simulink model "TST_CoETS_StTrqLimCalc"  (R2016b)
settings: Solver=FixedStepDiscrete  StartTime=0.0  StopTime=simTime  FixedStep=sampleTime  RelTol=1e-3
values from neighbouring files (symbols this model uses):
  testCase = 1    [initTST_CoETS_StTrqLimCalc_001.m]    (also in initTST_CoETS_StTrqLimCalc_002.m = 2)
libraries: simulink x19, UnitTest_Lib x16
settings Model: Creator=zhengjinyan  LastModifiedBy=zhengjinyan
settings DebuggingCC: SignalRangeChecking=error

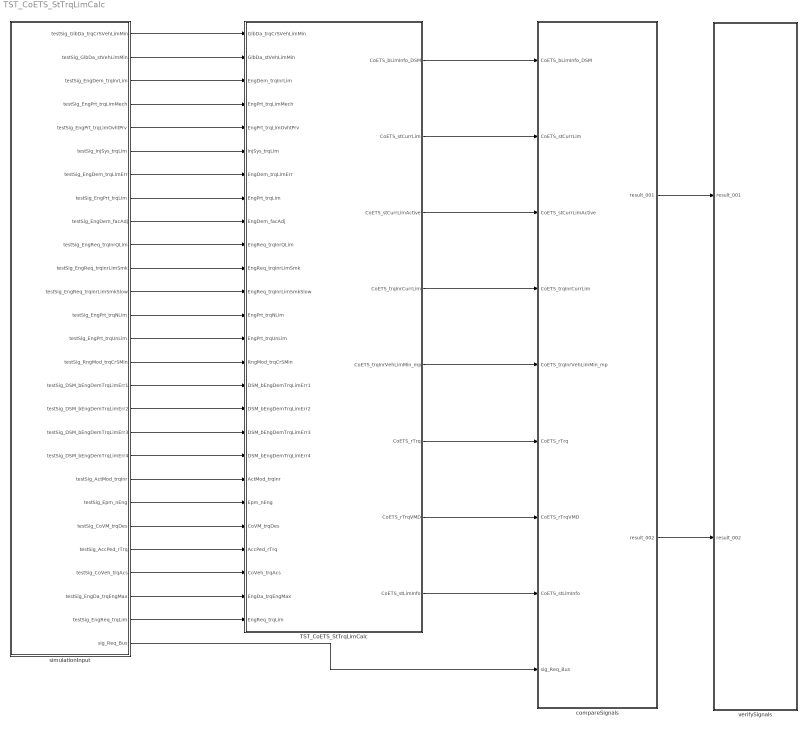
== system TST_CoETS_StTrqLimCalc ==
  TST_CoETS_StTrqLimCalc : Subsystem
  compareSignals : Subsystem
  simulationInput : Subsystem
  verifySignals : Subsystem
  wires:
  simulationInput/1(testSig_GlbDa_trqCrSVehLimMin) -> TST_CoETS_StTrqLimCalc/1(GlbDa_trqCrSVehLimMin)
  simulationInput/2(testSig_GlbDa_stVehLimMin) -> TST_CoETS_StTrqLimCalc/2(GlbDa_stVehLimMin)
  simulationInput/3(testSig_EngDem_trqInrLim) -> TST_CoETS_StTrqLimCalc/3(EngDem_trqInrLim)
  simulationInput/4(testSig_EngPrt_trqLimMech) -> TST_CoETS_StTrqLimCalc/4(EngPrt_trqLimMech)
  simulationInput/5(testSig_EngPrt_trqLimOvhtPrv) -> TST_CoETS_StTrqLimCalc/5(EngPrt_trqLimOvhtPrv)
  simulationInput/6(testSig_InjSys_trqLim) -> TST_CoETS_StTrqLimCalc/6(InjSys_trqLim)
  simulationInput/7(testSig_EngDem_trqLimErr) -> TST_CoETS_StTrqLimCalc/7(EngDem_trqLimErr)
  simulationInput/8(testSig_EngPrt_trqLim) -> TST_CoETS_StTrqLimCalc/8(EngPrt_trqLim)
  simulationInput/9(testSig_EngDem_facAdj) -> TST_CoETS_StTrqLimCalc/9(EngDem_facAdj)
  simulationInput/10(testSig_EngReq_trqInrQLim) -> TST_CoETS_StTrqLimCalc/10(EngReq_trqInrQLim)
  simulationInput/11(testSig_EngReq_trqInrLimSmk) -> TST_CoETS_StTrqLimCalc/11(EngReq_trqInrLimSmk)
  simulationInput/12(testSig_EngReq_trqInrLimSmkSlow) -> TST_CoETS_StTrqLimCalc/12(EngReq_trqInrLimSmkSlow)
  simulationInput/13(testSig_EngPrt_trqNLim) -> TST_CoETS_StTrqLimCalc/13(EngPrt_trqNLim)
  simulationInput/14(testSig_EngPrt_trqUnLim) -> TST_CoETS_StTrqLimCalc/14(EngPrt_trqUnLim)
  simulationInput/15(testSig_RngMod_trqCrSMin) -> TST_CoETS_StTrqLimCalc/15(RngMod_trqCrSMin)
  simulationInput/16(testSig_DSM_bEngDemTrqLimErr1) -> TST_CoETS_StTrqLimCalc/16(DSM_bEngDemTrqLimErr1)
  simulationInput/17(testSig_DSM_bEngDemTrqLimErr2) -> TST_CoETS_StTrqLimCalc/17(DSM_bEngDemTrqLimErr2)
  simulationInput/18(testSig_DSM_bEngDemTrqLimErr3) -> TST_CoETS_StTrqLimCalc/18(DSM_bEngDemTrqLimErr3)
  simulationInput/19(testSig_DSM_bEngDemTrqLimErr4) -> TST_CoETS_StTrqLimCalc/19(DSM_bEngDemTrqLimErr4)
  simulationInput/20(testSig_ActMod_trqInr) -> TST_CoETS_StTrqLimCalc/20(ActMod_trqInr)
  simulationInput/21(testSig_Epm_nEng) -> TST_CoETS_StTrqLimCalc/21(Epm_nEng)
  simulationInput/22(testSig_CoVM_trqDes) -> TST_CoETS_StTrqLimCalc/22(CoVM_trqDes)
  simulationInput/23(testSig_AccPed_rTrq) -> TST_CoETS_StTrqLimCalc/23(AccPed_rTrq)
  simulationInput/24(testSig_CoVeh_trqAcs) -> TST_CoETS_StTrqLimCalc/24(CoVeh_trqAcs)
  simulationInput/25(testSig_EngDa_trqEngMax) -> TST_CoETS_StTrqLimCalc/25(EngDa_trqEngMax)
  simulationInput/26(testSig_EngReq_trqLim) -> TST_CoETS_StTrqLimCalc/26(EngReq_trqLim)
  TST_CoETS_StTrqLimCalc/1(CoETS_bLimInfo_DSM) -> compareSignals/1(CoETS_bLimInfo_DSM)
  TST_CoETS_StTrqLimCalc/2(CoETS_stCurrLim) -> compareSignals/2(CoETS_stCurrLim)
  TST_CoETS_StTrqLimCalc/3(CoETS_stCurrLimActive) -> compareSignals/3(CoETS_stCurrLimActive)
  TST_CoETS_StTrqLimCalc/4(CoETS_trqInrCurrLim) -> compareSignals/4(CoETS_trqInrCurrLim)
  TST_CoETS_StTrqLimCalc/5(CoETS_trqInrVehLimMin_mp) -> compareSignals/5(CoETS_trqInrVehLimMin_mp)
  TST_CoETS_StTrqLimCalc/6(CoETS_rTrq) -> compareSignals/6(CoETS_rTrq)
  TST_CoETS_StTrqLimCalc/7(CoETS_rTrqVMD) -> compareSignals/7(CoETS_rTrqVMD)
  TST_CoETS_StTrqLimCalc/8(CoETS_stLimInfo) -> compareSignals/8(CoETS_stLimInfo)
  simulationInput/27(sig_Req_Bus) -> compareSignals/9(sig_Req_Bus)
  compareSignals/1(result_001) -> verifySignals/1(result_001)
  compareSignals/2(result_002) -> verifySignals/2(result_002)

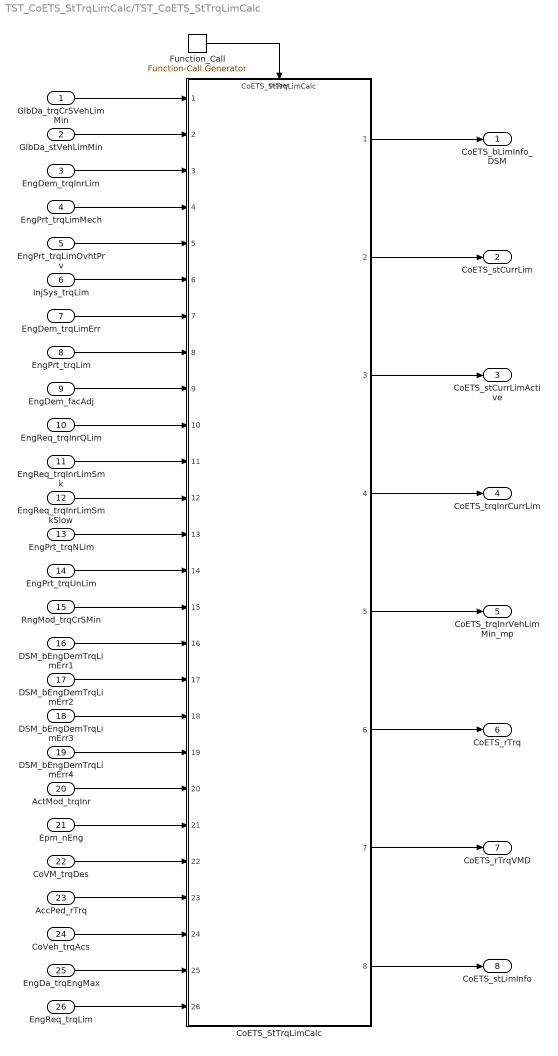
== system TST_CoETS_StTrqLimCalc/TST_CoETS_StTrqLimCalc ==
  GlbDa_trqCrSVehLimMin : Inport
  GlbDa_stVehLimMin : Inport  Port=2
  EngDem_trqInrLim : Inport  Port=3
  EngPrt_trqLimMech : Inport  Port=4
  EngPrt_trqLimOvhtPrv : Inport  Port=5
  InjSys_trqLim : Inport  Port=6
  EngDem_trqLimErr : Inport  Port=7
  EngPrt_trqLim : Inport  Port=8
  EngDem_facAdj : Inport  Port=9
  EngReq_trqInrQLim : Inport  Port=10
  EngReq_trqInrLimSmk : Inport  Port=11
  EngReq_trqInrLimSmkSlow : Inport  Port=12
  EngPrt_trqNLim : Inport  Port=13
  EngPrt_trqUnLim : Inport  Port=14
  RngMod_trqCrSMin : Inport  Port=15
  DSM_bEngDemTrqLimErr1 : Inport  Port=16
  DSM_bEngDemTrqLimErr2 : Inport  Port=17
  DSM_bEngDemTrqLimErr3 : Inport  Port=18
  DSM_bEngDemTrqLimErr4 : Inport  Port=19
  ActMod_trqInr : Inport  Port=20
  Epm_nEng : Inport  Port=21
  CoVM_trqDes : Inport  Port=22
  AccPed_rTrq : Inport  Port=23
  CoVeh_trqAcs : Inport  Port=24
  EngDa_trqEngMax : Inport  Port=25
  EngReq_trqLim : Inport  Port=26
  CoETS_StTrqLimCalc : ModelReference  ModelNameDialog=CoETS_StTrqLimCalc  SimulationMode=Normal  ModelReferenceVersion=1.4  TriggerPortName=function  TriggerPortTriggerType=function-call  TriggerPortStatesWhenEnabling=held
  Function_Call : simulink/Ports & Subsystems/Function-Call Generator  sample_time=sampleTime  numberOfIterations=1
  CoETS_bLimInfo_DSM : Outport
  CoETS_stCurrLim : Outport  Port=2
  CoETS_stCurrLimActive : Outport  Port=3
  CoETS_trqInrCurrLim : Outport  Port=4
  CoETS_trqInrVehLimMin_mp : Outport  Port=5
  CoETS_rTrq : Outport  Port=6
  CoETS_rTrqVMD : Outport  Port=7
  CoETS_stLimInfo : Outport  Port=8
  wires:
  Function_Call/1 -> CoETS_StTrqLimCalc/Trigger
  GlbDa_trqCrSVehLimMin/1 -> CoETS_StTrqLimCalc/1
  GlbDa_stVehLimMin/1 -> CoETS_StTrqLimCalc/2
  EngDem_trqInrLim/1 -> CoETS_StTrqLimCalc/3
  EngPrt_trqLimMech/1 -> CoETS_StTrqLimCalc/4
  EngPrt_trqLimOvhtPrv/1 -> CoETS_StTrqLimCalc/5
  InjSys_trqLim/1 -> CoETS_StTrqLimCalc/6
  EngDem_trqLimErr/1 -> CoETS_StTrqLimCalc/7
  EngPrt_trqLim/1 -> CoETS_StTrqLimCalc/8
  EngDem_facAdj/1 -> CoETS_StTrqLimCalc/9
  EngReq_trqInrQLim/1 -> CoETS_StTrqLimCalc/10
  EngReq_trqInrLimSmk/1 -> CoETS_StTrqLimCalc/11
  EngReq_trqInrLimSmkSlow/1 -> CoETS_StTrqLimCalc/12
  EngPrt_trqNLim/1 -> CoETS_StTrqLimCalc/13
  EngPrt_trqUnLim/1 -> CoETS_StTrqLimCalc/14
  RngMod_trqCrSMin/1 -> CoETS_StTrqLimCalc/15
  DSM_bEngDemTrqLimErr1/1 -> CoETS_StTrqLimCalc/16
  DSM_bEngDemTrqLimErr2/1 -> CoETS_StTrqLimCalc/17
  DSM_bEngDemTrqLimErr3/1 -> CoETS_StTrqLimCalc/18
  DSM_bEngDemTrqLimErr4/1 -> CoETS_StTrqLimCalc/19
  ActMod_trqInr/1 -> CoETS_StTrqLimCalc/20
  Epm_nEng/1 -> CoETS_StTrqLimCalc/21
  CoVM_trqDes/1 -> CoETS_StTrqLimCalc/22
  AccPed_rTrq/1 -> CoETS_StTrqLimCalc/23
  CoVeh_trqAcs/1 -> CoETS_StTrqLimCalc/24
  EngDa_trqEngMax/1 -> CoETS_StTrqLimCalc/25
  EngReq_trqLim/1 -> CoETS_StTrqLimCalc/26
  CoETS_StTrqLimCalc/1 -> CoETS_bLimInfo_DSM/1
  CoETS_StTrqLimCalc/2 -> CoETS_stCurrLim/1
  CoETS_StTrqLimCalc/3 -> CoETS_stCurrLimActive/1
  CoETS_StTrqLimCalc/4 -> CoETS_trqInrCurrLim/1
  CoETS_StTrqLimCalc/5 -> CoETS_trqInrVehLimMin_mp/1
  CoETS_StTrqLimCalc/6 -> CoETS_rTrq/1
  CoETS_StTrqLimCalc/7 -> CoETS_rTrqVMD/1
  CoETS_StTrqLimCalc/8 -> CoETS_stLimInfo/1

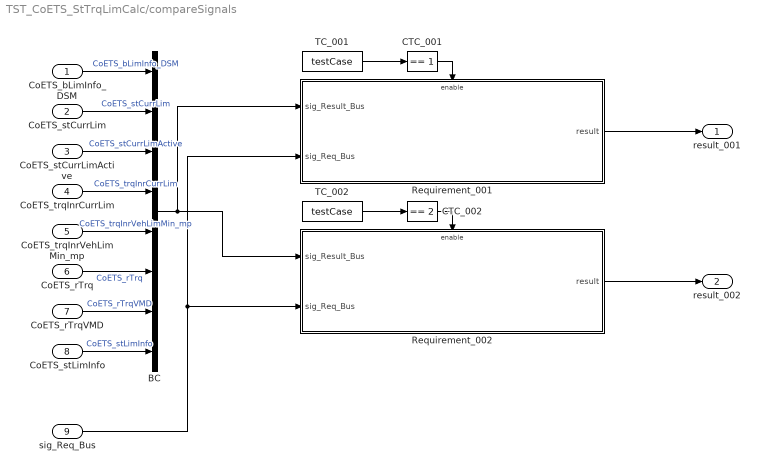
== system TST_CoETS_StTrqLimCalc/compareSignals ==
  CoETS_bLimInfo_DSM : Inport
  CoETS_stCurrLim : Inport  Port=2
  CoETS_stCurrLimActive : Inport  Port=3
  CoETS_trqInrCurrLim : Inport  Port=4
  CoETS_trqInrVehLimMin_mp : Inport  Port=5
  CoETS_rTrq : Inport  Port=6
  CoETS_rTrqVMD : Inport  Port=7
  CoETS_stLimInfo : Inport  Port=8
  sig_Req_Bus : Inport  Port=9
  BC : BusCreator  Inputs=8
  CTC_001 : simulink/Logic and Bit Operations/Compare To Constant  relop===  const=1  OutDataTypeStr=boolean
  CTC_002 : simulink/Logic and Bit Operations/Compare To Constant  relop===  const=2  OutDataTypeStr=boolean
  Requirement_001 : Subsystem
  Requirement_002 : Subsystem
  TC_001 : Constant  Value=testCase
  TC_002 : Constant  Value=testCase
  result_001 : Outport
  result_002 : Outport  Port=2
  wires:
  CoETS_bLimInfo_DSM/1 -> BC/1  "CoETS_bLimInfo_DSM"
  CoETS_stCurrLim/1 -> BC/2  "CoETS_stCurrLim"
  CoETS_stCurrLimActive/1 -> BC/3  "CoETS_stCurrLimActive"
  CoETS_trqInrCurrLim/1 -> BC/4  "CoETS_trqInrCurrLim"
  CoETS_trqInrVehLimMin_mp/1 -> BC/5  "CoETS_trqInrVehLimMin_mp"
  CoETS_rTrq/1 -> BC/6  "CoETS_rTrq"
  CoETS_rTrqVMD/1 -> BC/7  "CoETS_rTrqVMD"
  CoETS_stLimInfo/1 -> BC/8  "CoETS_stLimInfo"
  TC_001/1 -> CTC_001/1
  CTC_001/1 -> Requirement_001/Enable
  sig_Req_Bus/1 -> Requirement_001/2(sig_Req_Bus), Requirement_002/2(sig_Req_Bus)
  BC/1 -> Requirement_001/1(sig_Result_Bus), Requirement_002/1(sig_Result_Bus)
  Requirement_001/1(result) -> result_001/1
  TC_002/1 -> CTC_002/1
  CTC_002/1 -> Requirement_002/Enable
  Requirement_002/1(result) -> result_002/1

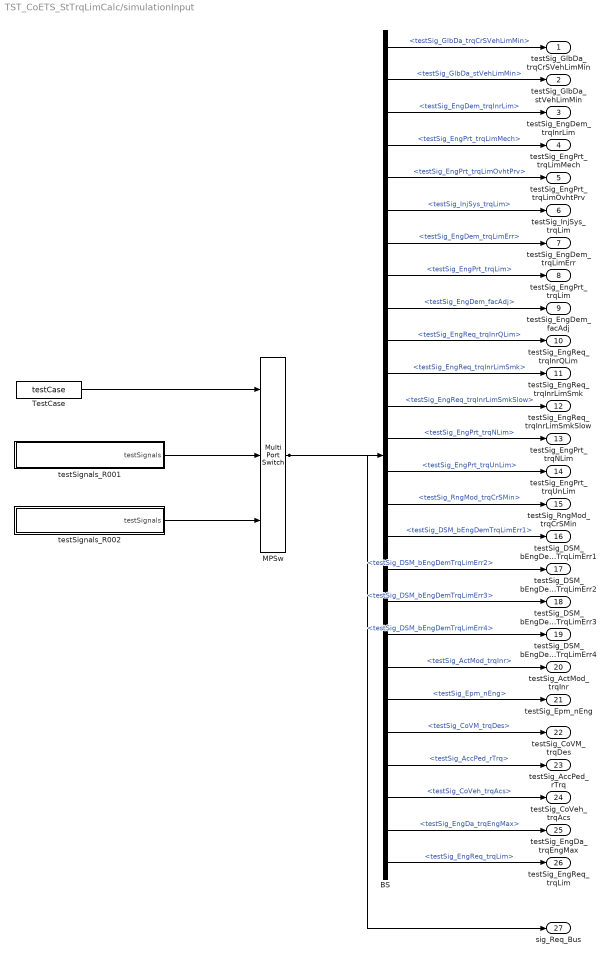
== system TST_CoETS_StTrqLimCalc/simulationInput ==
  BS : BusSelector  OutputSignals=testSig_GlbDa_trqCrSVehLimMin,testSig_GlbDa_stVehLimMin,testSig_EngDem_trqInrLim,testSig_EngPrt_trqLimMech,testSig_EngPrt_trqLimOvhtPrv,testSig_InjSys_trqLim,testSig_EngDem_trqLimErr,testSig_EngPrt_trqLim,testSig_EngDem_facAdj,testSig_EngReq_trqInrQLim,testSig_EngReq_trqInrLimSmk,testSig_EngReq_trqInrLimSmkSlow,testSig_EngPrt_trqNLim,testSig_EngPrt_trqUnLim,testSig_RngMod_trqCrSMin,testSig_DSM_bEngDemTrqLimErr1,testSig_DSM_bEngDemTrqLimErr2,testSig_DSM_bEngDemTrqLimErr3,testSig_DSM_bEngDemTrqLimErr4,testSig_ActMod_trqInr,testSig_Epm_nEng,testSig_CoVM_trqDes,testSig_AccPed_rTrq,testSig_CoVeh_trqAcs,testSig_EngDa_trqEngMax,testSig_EngReq_trqLim
  MPSw : MultiPortSwitch  Inputs=2  SaturateOnIntegerOverflow=on  InputSameDT=on
  TestCase : Constant  Value=testCase
  testSignals_R001 : Subsystem
  testSignals_R002 : Subsystem
  testSig_GlbDa_trqCrSVehLimMin : Outport
  testSig_GlbDa_stVehLimMin : Outport  Port=2
  testSig_EngDem_trqInrLim : Outport  Port=3
  testSig_EngPrt_trqLimMech : Outport  Port=4
  testSig_EngPrt_trqLimOvhtPrv : Outport  Port=5
  testSig_InjSys_trqLim : Outport  Port=6
  testSig_EngDem_trqLimErr : Outport  Port=7
  testSig_EngPrt_trqLim : Outport  Port=8
  testSig_EngDem_facAdj : Outport  Port=9
  testSig_EngReq_trqInrQLim : Outport  Port=10
  testSig_EngReq_trqInrLimSmk : Outport  Port=11
  testSig_EngReq_trqInrLimSmkSlow : Outport  Port=12
  testSig_EngPrt_trqNLim : Outport  Port=13
  testSig_EngPrt_trqUnLim : Outport  Port=14
  testSig_RngMod_trqCrSMin : Outport  Port=15
  testSig_DSM_bEngDemTrqLimErr1 : Outport  Port=16
  testSig_DSM_bEngDemTrqLimErr2 : Outport  Port=17
  testSig_DSM_bEngDemTrqLimErr3 : Outport  Port=18
  testSig_DSM_bEngDemTrqLimErr4 : Outport  Port=19
  testSig_ActMod_trqInr : Outport  Port=20
  testSig_Epm_nEng : Outport  Port=21
  testSig_CoVM_trqDes : Outport  Port=22
  testSig_AccPed_rTrq : Outport  Port=23
  testSig_CoVeh_trqAcs : Outport  Port=24
  testSig_EngDa_trqEngMax : Outport  Port=25
  testSig_EngReq_trqLim : Outport  Port=26
  sig_Req_Bus : Outport  Port=27
  wires:
  BS/1 -> testSig_GlbDa_trqCrSVehLimMin/1  "<testSig_GlbDa_trqCrSVehLimMin>"
  BS/2 -> testSig_GlbDa_stVehLimMin/1  "<testSig_GlbDa_stVehLimMin>"
  BS/3 -> testSig_EngDem_trqInrLim/1  "<testSig_EngDem_trqInrLim>"
  BS/4 -> testSig_EngPrt_trqLimMech/1  "<testSig_EngPrt_trqLimMech>"
  BS/5 -> testSig_EngPrt_trqLimOvhtPrv/1  "<testSig_EngPrt_trqLimOvhtPrv>"
  BS/6 -> testSig_InjSys_trqLim/1  "<testSig_InjSys_trqLim>"
  BS/7 -> testSig_EngDem_trqLimErr/1  "<testSig_EngDem_trqLimErr>"
  BS/8 -> testSig_EngPrt_trqLim/1  "<testSig_EngPrt_trqLim>"
  BS/9 -> testSig_EngDem_facAdj/1  "<testSig_EngDem_facAdj>"
  BS/10 -> testSig_EngReq_trqInrQLim/1  "<testSig_EngReq_trqInrQLim>"
  BS/11 -> testSig_EngReq_trqInrLimSmk/1  "<testSig_EngReq_trqInrLimSmk>"
  BS/12 -> testSig_EngReq_trqInrLimSmkSlow/1  "<testSig_EngReq_trqInrLimSmkSlow>"
  BS/13 -> testSig_EngPrt_trqNLim/1  "<testSig_EngPrt_trqNLim>"
  BS/14 -> testSig_EngPrt_trqUnLim/1  "<testSig_EngPrt_trqUnLim>"
  BS/15 -> testSig_RngMod_trqCrSMin/1  "<testSig_RngMod_trqCrSMin>"
  BS/16 -> testSig_DSM_bEngDemTrqLimErr1/1  "<testSig_DSM_bEngDemTrqLimErr1>"
  BS/17 -> testSig_DSM_bEngDemTrqLimErr2/1  "<testSig_DSM_bEngDemTrqLimErr2>"
  BS/18 -> testSig_DSM_bEngDemTrqLimErr3/1  "<testSig_DSM_bEngDemTrqLimErr3>"
  BS/19 -> testSig_DSM_bEngDemTrqLimErr4/1  "<testSig_DSM_bEngDemTrqLimErr4>"
  BS/20 -> testSig_ActMod_trqInr/1  "<testSig_ActMod_trqInr>"
  BS/21 -> testSig_Epm_nEng/1  "<testSig_Epm_nEng>"
  BS/22 -> testSig_CoVM_trqDes/1  "<testSig_CoVM_trqDes>"
  BS/23 -> testSig_AccPed_rTrq/1  "<testSig_AccPed_rTrq>"
  BS/24 -> testSig_CoVeh_trqAcs/1  "<testSig_CoVeh_trqAcs>"
  BS/25 -> testSig_EngDa_trqEngMax/1  "<testSig_EngDa_trqEngMax>"
  BS/26 -> testSig_EngReq_trqLim/1  "<testSig_EngReq_trqLim>"
  MPSw/1 -> BS/1, sig_Req_Bus/1
  TestCase/1 -> MPSw/1
  testSignals_R001/1(testSignals) -> MPSw/2
  testSignals_R002/1(testSignals) -> MPSw/3

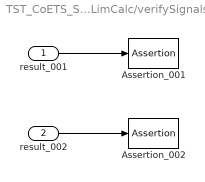
== system TST_CoETS_StTrqLimCalc/verifySignals ==
  result_001 : Inport
  result_002 : Inport  Port=2
  Assertion_001 : Assertion  Enabled=off
  Assertion_002 : Assertion  Enabled=off
  wires:
  result_001/1 -> Assertion_001/1
  result_002/1 -> Assertion_002/1

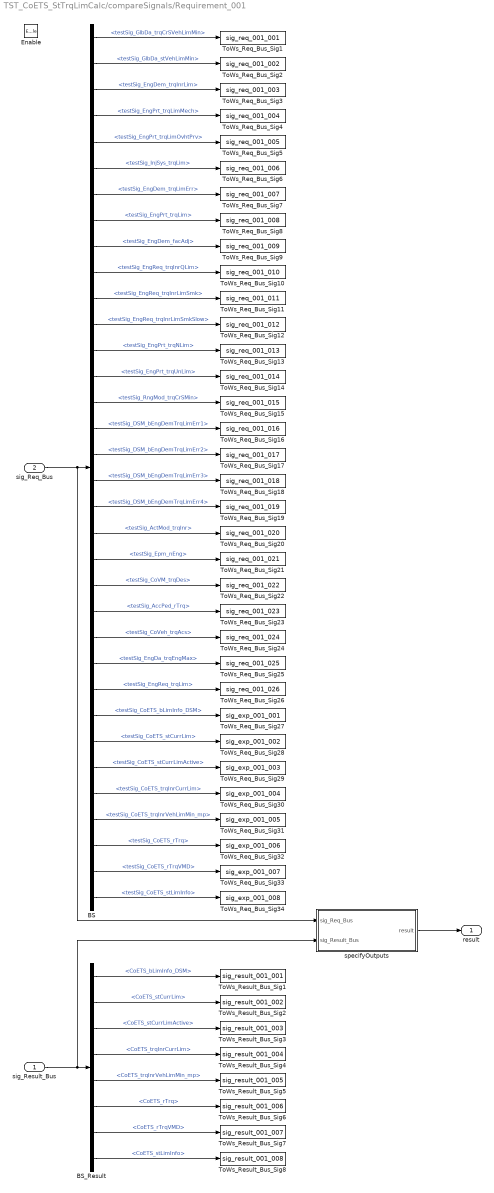
== system TST_CoETS_StTrqLimCalc/compareSignals/Requirement_001 ==
  sig_Result_Bus : Inport
  sig_Req_Bus : Inport  Port=2
  Enable : EnablePort
  BS : BusSelector  OutputSignals=testSig_GlbDa_trqCrSVehLimMin,testSig_GlbDa_stVehLimMin,testSig_EngDem_trqInrLim,testSig_EngPrt_trqLimMech,testSig_EngPrt_trqLimOvhtPrv,testSig_InjSys_trqLim,testSig_EngDem_trqLimErr,testSig_EngPrt_trqLim,testSig_EngDem_facAdj,testSig_EngReq_trqInrQLim,testSig_EngReq_trqInrLimSmk,testSig_EngReq_trqInrLimSmkSlow,testSig_EngPrt_trqNLim,testSig_EngPrt_trqUnLim,testSig_RngMod_trqCrSMin,testSig_DSM_bEngDemTrqLimErr1,testSig_DSM_bEngDemTrqLimErr2,testSig_DSM_bEngDemTrqLimErr3,testSig_DSM_bEngDemTrqLimErr4,testSig_ActMod_trqInr,testSig_Epm_nEng,testSig_CoVM_trqDes,testSig_AccPed_rTrq,testSig_CoVeh_trqAcs,testSig_EngDa_trqEngMax,testSig_EngReq_trqLim,testSig_CoETS_bLimInfo_DSM,testSig_CoETS_stCurrLim,testSig_CoETS_stCurrLimActive,testSig_CoETS_trqInrCurrLim,testSig_CoETS_trqInrVehLimMin_mp,testSig_CoETS_rTrq,testSig_CoETS_rTrqVMD,testSig_CoETS_stLimInfo
  BS_Result : BusSelector  OutputSignals=CoETS_bLimInfo_DSM,CoETS_stCurrLim,CoETS_stCurrLimActive,CoETS_trqInrCurrLim,CoETS_trqInrVehLimMin_mp,CoETS_rTrq,CoETS_rTrqVMD,CoETS_stLimInfo
  ToWs_Req_Bus_Sig1 : ToWorkspace  VariableName=sig_req_001_001  SaveFormat=Structure With Time
  ToWs_Req_Bus_Sig10 : ToWorkspace  VariableName=sig_req_001_010  SaveFormat=Structure With Time
  ToWs_Req_Bus_Sig11 : ToWorkspace  VariableName=sig_req_001_011  SaveFormat=Structure With Time
  ToWs_Req_Bus_Sig12 : ToWorkspace  VariableName=sig_req_001_012  SaveFormat=Structure With Time
  ToWs_Req_Bus_Sig13 : ToWorkspace  VariableName=sig_req_001_013  SaveFormat=Structure With Time
  ToWs_Req_Bus_Sig14 : ToWorkspace  VariableName=sig_req_001_014  SaveFormat=Structure With Time
  ToWs_Req_Bus_Sig15 : ToWorkspace  VariableName=sig_req_001_015  SaveFormat=Structure With Time
  ToWs_Req_Bus_Sig16 : ToWorkspace  VariableName=sig_req_001_016  SaveFormat=Structure With Time
  ToWs_Req_Bus_Sig17 : ToWorkspace  VariableName=sig_req_001_017  SaveFormat=Structure With Time
  ToWs_Req_Bus_Sig18 : ToWorkspace  VariableName=sig_req_001_018  SaveFormat=Structure With Time
  ToWs_Req_Bus_Sig19 : ToWorkspace  VariableName=sig_req_001_019  SaveFormat=Structure With Time
  ToWs_Req_Bus_Sig2 : ToWorkspace  VariableName=sig_req_001_002  SaveFormat=Structure With Time
  ToWs_Req_Bus_Sig20 : ToWorkspace  VariableName=sig_req_001_020  SaveFormat=Structure With Time
  ToWs_Req_Bus_Sig21 : ToWorkspace  VariableName=sig_req_001_021  SaveFormat=Structure With Time
  ToWs_Req_Bus_Sig22 : ToWorkspace  VariableName=sig_req_001_022  SaveFormat=Structure With Time
  ToWs_Req_Bus_Sig23 : ToWorkspace  VariableName=sig_req_001_023  SaveFormat=Structure With Time
  ToWs_Req_Bus_Sig24 : ToWorkspace  VariableName=sig_req_001_024  SaveFormat=Structure With Time
  ToWs_Req_Bus_Sig25 : ToWorkspace  VariableName=sig_req_001_025  SaveFormat=Structure With Time
  ToWs_Req_Bus_Sig26 : ToWorkspace  VariableName=sig_req_001_026  SaveFormat=Structure With Time
  ToWs_Req_Bus_Sig27 : ToWorkspace  VariableName=sig_exp_001_001  SaveFormat=Structure With Time
  ToWs_Req_Bus_Sig28 : ToWorkspace  VariableName=sig_exp_001_002  SaveFormat=Structure With Time
  ToWs_Req_Bus_Sig29 : ToWorkspace  VariableName=sig_exp_001_003  SaveFormat=Structure With Time
  ToWs_Req_Bus_Sig3 : ToWorkspace  VariableName=sig_req_001_003  SaveFormat=Structure With Time
  ToWs_Req_Bus_Sig30 : ToWorkspace  VariableName=sig_exp_001_004  SaveFormat=Structure With Time
  ToWs_Req_Bus_Sig31 : ToWorkspace  VariableName=sig_exp_001_005  SaveFormat=Structure With Time
  ToWs_Req_Bus_Sig32 : ToWorkspace  VariableName=sig_exp_001_006  SaveFormat=Structure With Time
  ToWs_Req_Bus_Sig33 : ToWorkspace  VariableName=sig_exp_001_007  SaveFormat=Structure With Time
  ToWs_Req_Bus_Sig34 : ToWorkspace  VariableName=sig_exp_001_008  SaveFormat=Structure With Time
  ToWs_Req_Bus_Sig4 : ToWorkspace  VariableName=sig_req_001_004  SaveFormat=Structure With Time
  ToWs_Req_Bus_Sig5 : ToWorkspace  VariableName=sig_req_001_005  SaveFormat=Structure With Time
  ToWs_Req_Bus_Sig6 : ToWorkspace  VariableName=sig_req_001_006  SaveFormat=Structure With Time
  ToWs_Req_Bus_Sig7 : ToWorkspace  VariableName=sig_req_001_007  SaveFormat=Structure With Time
  ToWs_Req_Bus_Sig8 : ToWorkspace  VariableName=sig_req_001_008  SaveFormat=Structure With Time
  ToWs_Req_Bus_Sig9 : ToWorkspace  VariableName=sig_req_001_009  SaveFormat=Structure With Time
  ToWs_Result_Bus_Sig1 : ToWorkspace  VariableName=sig_result_001_001  SaveFormat=Structure With Time
  ToWs_Result_Bus_Sig2 : ToWorkspace  VariableName=sig_result_001_002  SaveFormat=Structure With Time
  ToWs_Result_Bus_Sig3 : ToWorkspace  VariableName=sig_result_001_003  SaveFormat=Structure With Time
  ToWs_Result_Bus_Sig4 : ToWorkspace  VariableName=sig_result_001_004  SaveFormat=Structure With Time
  ToWs_Result_Bus_Sig5 : ToWorkspace  VariableName=sig_result_001_005  SaveFormat=Structure With Time
  ToWs_Result_Bus_Sig6 : ToWorkspace  VariableName=sig_result_001_006  SaveFormat=Structure With Time
  ToWs_Result_Bus_Sig7 : ToWorkspace  VariableName=sig_result_001_007  SaveFormat=Structure With Time
  ToWs_Result_Bus_Sig8 : ToWorkspace  VariableName=sig_result_001_008  SaveFormat=Structure With Time
  specifyOutputs : Subsystem
  result : Outport
  wires:
  sig_Req_Bus/1 -> BS/1, specifyOutputs/1(sig_Req_Bus)
  BS/1 -> ToWs_Req_Bus_Sig1/1  "<testSig_GlbDa_trqCrSVehLimMin>"
  BS/2 -> ToWs_Req_Bus_Sig2/1  "<testSig_GlbDa_stVehLimMin>"
  BS/3 -> ToWs_Req_Bus_Sig3/1  "<testSig_EngDem_trqInrLim>"
  BS/4 -> ToWs_Req_Bus_Sig4/1  "<testSig_EngPrt_trqLimMech>"
  BS/5 -> ToWs_Req_Bus_Sig5/1  "<testSig_EngPrt_trqLimOvhtPrv>"
  BS/6 -> ToWs_Req_Bus_Sig6/1  "<testSig_InjSys_trqLim>"
  BS/7 -> ToWs_Req_Bus_Sig7/1  "<testSig_EngDem_trqLimErr>"
  BS/8 -> ToWs_Req_Bus_Sig8/1  "<testSig_EngPrt_trqLim>"
  BS/9 -> ToWs_Req_Bus_Sig9/1  "<testSig_EngDem_facAdj>"
  BS/10 -> ToWs_Req_Bus_Sig10/1  "<testSig_EngReq_trqInrQLim>"
  BS/11 -> ToWs_Req_Bus_Sig11/1  "<testSig_EngReq_trqInrLimSmk>"
  BS/12 -> ToWs_Req_Bus_Sig12/1  "<testSig_EngReq_trqInrLimSmkSlow>"
  BS/13 -> ToWs_Req_Bus_Sig13/1  "<testSig_EngPrt_trqNLim>"
  BS/14 -> ToWs_Req_Bus_Sig14/1  "<testSig_EngPrt_trqUnLim>"
  BS/15 -> ToWs_Req_Bus_Sig15/1  "<testSig_RngMod_trqCrSMin>"
  BS/16 -> ToWs_Req_Bus_Sig16/1  "<testSig_DSM_bEngDemTrqLimErr1>"
  BS/17 -> ToWs_Req_Bus_Sig17/1  "<testSig_DSM_bEngDemTrqLimErr2>"
  BS/18 -> ToWs_Req_Bus_Sig18/1  "<testSig_DSM_bEngDemTrqLimErr3>"
  BS/19 -> ToWs_Req_Bus_Sig19/1  "<testSig_DSM_bEngDemTrqLimErr4>"
  BS/20 -> ToWs_Req_Bus_Sig20/1  "<testSig_ActMod_trqInr>"
  BS/21 -> ToWs_Req_Bus_Sig21/1  "<testSig_Epm_nEng>"
  BS/22 -> ToWs_Req_Bus_Sig22/1  "<testSig_CoVM_trqDes>"
  BS/23 -> ToWs_Req_Bus_Sig23/1  "<testSig_AccPed_rTrq>"
  BS/24 -> ToWs_Req_Bus_Sig24/1  "<testSig_CoVeh_trqAcs>"
  BS/25 -> ToWs_Req_Bus_Sig25/1  "<testSig_EngDa_trqEngMax>"
  BS/26 -> ToWs_Req_Bus_Sig26/1  "<testSig_EngReq_trqLim>"
  BS/27 -> ToWs_Req_Bus_Sig27/1  "<testSig_CoETS_bLimInfo_DSM>"
  BS/28 -> ToWs_Req_Bus_Sig28/1  "<testSig_CoETS_stCurrLim>"
  BS/29 -> ToWs_Req_Bus_Sig29/1  "<testSig_CoETS_stCurrLimActive>"
  BS/30 -> ToWs_Req_Bus_Sig30/1  "<testSig_CoETS_trqInrCurrLim>"
  BS/31 -> ToWs_Req_Bus_Sig31/1  "<testSig_CoETS_trqInrVehLimMin_mp>"
  BS/32 -> ToWs_Req_Bus_Sig32/1  "<testSig_CoETS_rTrq>"
  BS/33 -> ToWs_Req_Bus_Sig33/1  "<testSig_CoETS_rTrqVMD>"
  BS/34 -> ToWs_Req_Bus_Sig34/1  "<testSig_CoETS_stLimInfo>"
  sig_Result_Bus/1 -> BS_Result/1, specifyOutputs/2(sig_Result_Bus)
  BS_Result/1 -> ToWs_Result_Bus_Sig1/1  "<CoETS_bLimInfo_DSM>"
  BS_Result/2 -> ToWs_Result_Bus_Sig2/1  "<CoETS_stCurrLim>"
  BS_Result/3 -> ToWs_Result_Bus_Sig3/1  "<CoETS_stCurrLimActive>"
  BS_Result/4 -> ToWs_Result_Bus_Sig4/1  "<CoETS_trqInrCurrLim>"
  BS_Result/5 -> ToWs_Result_Bus_Sig5/1  "<CoETS_trqInrVehLimMin_mp>"
  BS_Result/6 -> ToWs_Result_Bus_Sig6/1  "<CoETS_rTrq>"
  BS_Result/7 -> ToWs_Result_Bus_Sig7/1  "<CoETS_rTrqVMD>"
  BS_Result/8 -> ToWs_Result_Bus_Sig8/1  "<CoETS_stLimInfo>"
  specifyOutputs/1(result) -> result/1

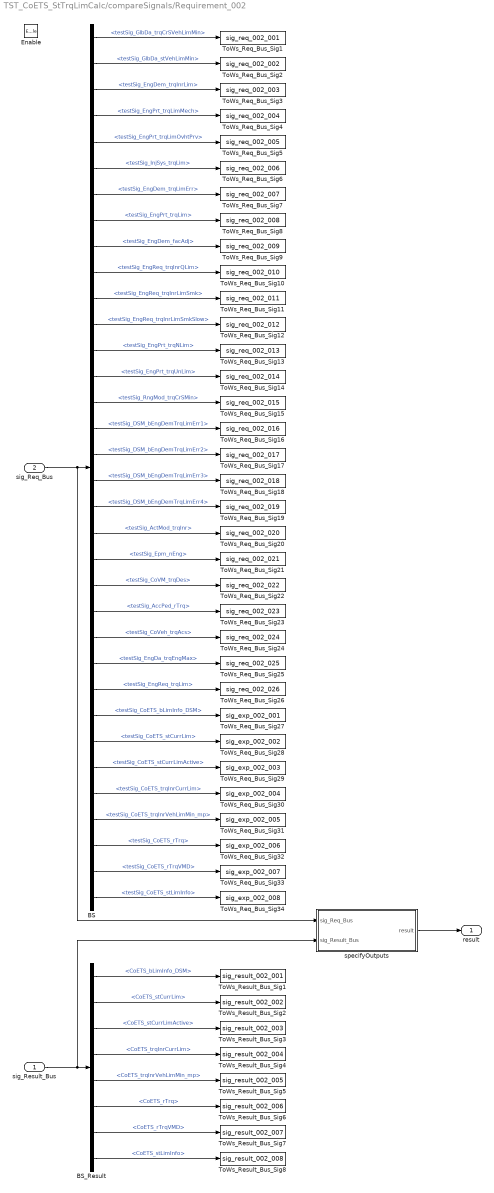
== system TST_CoETS_StTrqLimCalc/compareSignals/Requirement_002 ==
  sig_Result_Bus : Inport
  sig_Req_Bus : Inport  Port=2
  Enable : EnablePort
  BS : BusSelector  OutputSignals=testSig_GlbDa_trqCrSVehLimMin,testSig_GlbDa_stVehLimMin,testSig_EngDem_trqInrLim,testSig_EngPrt_trqLimMech,testSig_EngPrt_trqLimOvhtPrv,testSig_InjSys_trqLim,testSig_EngDem_trqLimErr,testSig_EngPrt_trqLim,testSig_EngDem_facAdj,testSig_EngReq_trqInrQLim,testSig_EngReq_trqInrLimSmk,testSig_EngReq_trqInrLimSmkSlow,testSig_EngPrt_trqNLim,testSig_EngPrt_trqUnLim,testSig_RngMod_trqCrSMin,testSig_DSM_bEngDemTrqLimErr1,testSig_DSM_bEngDemTrqLimErr2,testSig_DSM_bEngDemTrqLimErr3,testSig_DSM_bEngDemTrqLimErr4,testSig_ActMod_trqInr,testSig_Epm_nEng,testSig_CoVM_trqDes,testSig_AccPed_rTrq,testSig_CoVeh_trqAcs,testSig_EngDa_trqEngMax,testSig_EngReq_trqLim,testSig_CoETS_bLimInfo_DSM,testSig_CoETS_stCurrLim,testSig_CoETS_stCurrLimActive,testSig_CoETS_trqInrCurrLim,testSig_CoETS_trqInrVehLimMin_mp,testSig_CoETS_rTrq,testSig_CoETS_rTrqVMD,testSig_CoETS_stLimInfo
  BS_Result : BusSelector  OutputSignals=CoETS_bLimInfo_DSM,CoETS_stCurrLim,CoETS_stCurrLimActive,CoETS_trqInrCurrLim,CoETS_trqInrVehLimMin_mp,CoETS_rTrq,CoETS_rTrqVMD,CoETS_stLimInfo
  ToWs_Req_Bus_Sig1 : ToWorkspace  VariableName=sig_req_002_001  SaveFormat=Structure With Time
  ToWs_Req_Bus_Sig10 : ToWorkspace  VariableName=sig_req_002_010  SaveFormat=Structure With Time
  ToWs_Req_Bus_Sig11 : ToWorkspace  VariableName=sig_req_002_011  SaveFormat=Structure With Time
  ToWs_Req_Bus_Sig12 : ToWorkspace  VariableName=sig_req_002_012  SaveFormat=Structure With Time
  ToWs_Req_Bus_Sig13 : ToWorkspace  VariableName=sig_req_002_013  SaveFormat=Structure With Time
  ToWs_Req_Bus_Sig14 : ToWorkspace  VariableName=sig_req_002_014  SaveFormat=Structure With Time
  ToWs_Req_Bus_Sig15 : ToWorkspace  VariableName=sig_req_002_015  SaveFormat=Structure With Time
  ToWs_Req_Bus_Sig16 : ToWorkspace  VariableName=sig_req_002_016  SaveFormat=Structure With Time
  ToWs_Req_Bus_Sig17 : ToWorkspace  VariableName=sig_req_002_017  SaveFormat=Structure With Time
  ToWs_Req_Bus_Sig18 : ToWorkspace  VariableName=sig_req_002_018  SaveFormat=Structure With Time
  ToWs_Req_Bus_Sig19 : ToWorkspace  VariableName=sig_req_002_019  SaveFormat=Structure With Time
  ToWs_Req_Bus_Sig2 : ToWorkspace  VariableName=sig_req_002_002  SaveFormat=Structure With Time
  ToWs_Req_Bus_Sig20 : ToWorkspace  VariableName=sig_req_002_020  SaveFormat=Structure With Time
  ToWs_Req_Bus_Sig21 : ToWorkspace  VariableName=sig_req_002_021  SaveFormat=Structure With Time
  ToWs_Req_Bus_Sig22 : ToWorkspace  VariableName=sig_req_002_022  SaveFormat=Structure With Time
  ToWs_Req_Bus_Sig23 : ToWorkspace  VariableName=sig_req_002_023  SaveFormat=Structure With Time
  ToWs_Req_Bus_Sig24 : ToWorkspace  VariableName=sig_req_002_024  SaveFormat=Structure With Time
  ToWs_Req_Bus_Sig25 : ToWorkspace  VariableName=sig_req_002_025  SaveFormat=Structure With Time
  ToWs_Req_Bus_Sig26 : ToWorkspace  VariableName=sig_req_002_026  SaveFormat=Structure With Time
  ToWs_Req_Bus_Sig27 : ToWorkspace  VariableName=sig_exp_002_001  SaveFormat=Structure With Time
  ToWs_Req_Bus_Sig28 : ToWorkspace  VariableName=sig_exp_002_002  SaveFormat=Structure With Time
  ToWs_Req_Bus_Sig29 : ToWorkspace  VariableName=sig_exp_002_003  SaveFormat=Structure With Time
  ToWs_Req_Bus_Sig3 : ToWorkspace  VariableName=sig_req_002_003  SaveFormat=Structure With Time
  ToWs_Req_Bus_Sig30 : ToWorkspace  VariableName=sig_exp_002_004  SaveFormat=Structure With Time
  ToWs_Req_Bus_Sig31 : ToWorkspace  VariableName=sig_exp_002_005  SaveFormat=Structure With Time
  ToWs_Req_Bus_Sig32 : ToWorkspace  VariableName=sig_exp_002_006  SaveFormat=Structure With Time
  ToWs_Req_Bus_Sig33 : ToWorkspace  VariableName=sig_exp_002_007  SaveFormat=Structure With Time
  ToWs_Req_Bus_Sig34 : ToWorkspace  VariableName=sig_exp_002_008  SaveFormat=Structure With Time
  ToWs_Req_Bus_Sig4 : ToWorkspace  VariableName=sig_req_002_004  SaveFormat=Structure With Time
  ToWs_Req_Bus_Sig5 : ToWorkspace  VariableName=sig_req_002_005  SaveFormat=Structure With Time
  ToWs_Req_Bus_Sig6 : ToWorkspace  VariableName=sig_req_002_006  SaveFormat=Structure With Time
  ToWs_Req_Bus_Sig7 : ToWorkspace  VariableName=sig_req_002_007  SaveFormat=Structure With Time
  ToWs_Req_Bus_Sig8 : ToWorkspace  VariableName=sig_req_002_008  SaveFormat=Structure With Time
  ToWs_Req_Bus_Sig9 : ToWorkspace  VariableName=sig_req_002_009  SaveFormat=Structure With Time
  ToWs_Result_Bus_Sig1 : ToWorkspace  VariableName=sig_result_002_001  SaveFormat=Structure With Time
  ToWs_Result_Bus_Sig2 : ToWorkspace  VariableName=sig_result_002_002  SaveFormat=Structure With Time
  ToWs_Result_Bus_Sig3 : ToWorkspace  VariableName=sig_result_002_003  SaveFormat=Structure With Time
  ToWs_Result_Bus_Sig4 : ToWorkspace  VariableName=sig_result_002_004  SaveFormat=Structure With Time
  ToWs_Result_Bus_Sig5 : ToWorkspace  VariableName=sig_result_002_005  SaveFormat=Structure With Time
  ToWs_Result_Bus_Sig6 : ToWorkspace  VariableName=sig_result_002_006  SaveFormat=Structure With Time
  ToWs_Result_Bus_Sig7 : ToWorkspace  VariableName=sig_result_002_007  SaveFormat=Structure With Time
  ToWs_Result_Bus_Sig8 : ToWorkspace  VariableName=sig_result_002_008  SaveFormat=Structure With Time
  specifyOutputs : Subsystem
  result : Outport
  wires:
  sig_Req_Bus/1 -> BS/1, specifyOutputs/1(sig_Req_Bus)
  BS/1 -> ToWs_Req_Bus_Sig1/1  "<testSig_GlbDa_trqCrSVehLimMin>"
  BS/2 -> ToWs_Req_Bus_Sig2/1  "<testSig_GlbDa_stVehLimMin>"
  BS/3 -> ToWs_Req_Bus_Sig3/1  "<testSig_EngDem_trqInrLim>"
  BS/4 -> ToWs_Req_Bus_Sig4/1  "<testSig_EngPrt_trqLimMech>"
  BS/5 -> ToWs_Req_Bus_Sig5/1  "<testSig_EngPrt_trqLimOvhtPrv>"
  BS/6 -> ToWs_Req_Bus_Sig6/1  "<testSig_InjSys_trqLim>"
  BS/7 -> ToWs_Req_Bus_Sig7/1  "<testSig_EngDem_trqLimErr>"
  BS/8 -> ToWs_Req_Bus_Sig8/1  "<testSig_EngPrt_trqLim>"
  BS/9 -> ToWs_Req_Bus_Sig9/1  "<testSig_EngDem_facAdj>"
  BS/10 -> ToWs_Req_Bus_Sig10/1  "<testSig_EngReq_trqInrQLim>"
  BS/11 -> ToWs_Req_Bus_Sig11/1  "<testSig_EngReq_trqInrLimSmk>"
  BS/12 -> ToWs_Req_Bus_Sig12/1  "<testSig_EngReq_trqInrLimSmkSlow>"
  BS/13 -> ToWs_Req_Bus_Sig13/1  "<testSig_EngPrt_trqNLim>"
  BS/14 -> ToWs_Req_Bus_Sig14/1  "<testSig_EngPrt_trqUnLim>"
  BS/15 -> ToWs_Req_Bus_Sig15/1  "<testSig_RngMod_trqCrSMin>"
  BS/16 -> ToWs_Req_Bus_Sig16/1  "<testSig_DSM_bEngDemTrqLimErr1>"
  BS/17 -> ToWs_Req_Bus_Sig17/1  "<testSig_DSM_bEngDemTrqLimErr2>"
  BS/18 -> ToWs_Req_Bus_Sig18/1  "<testSig_DSM_bEngDemTrqLimErr3>"
  BS/19 -> ToWs_Req_Bus_Sig19/1  "<testSig_DSM_bEngDemTrqLimErr4>"
  BS/20 -> ToWs_Req_Bus_Sig20/1  "<testSig_ActMod_trqInr>"
  BS/21 -> ToWs_Req_Bus_Sig21/1  "<testSig_Epm_nEng>"
  BS/22 -> ToWs_Req_Bus_Sig22/1  "<testSig_CoVM_trqDes>"
  BS/23 -> ToWs_Req_Bus_Sig23/1  "<testSig_AccPed_rTrq>"
  BS/24 -> ToWs_Req_Bus_Sig24/1  "<testSig_CoVeh_trqAcs>"
  BS/25 -> ToWs_Req_Bus_Sig25/1  "<testSig_EngDa_trqEngMax>"
  BS/26 -> ToWs_Req_Bus_Sig26/1  "<testSig_EngReq_trqLim>"
  BS/27 -> ToWs_Req_Bus_Sig27/1  "<testSig_CoETS_bLimInfo_DSM>"
  BS/28 -> ToWs_Req_Bus_Sig28/1  "<testSig_CoETS_stCurrLim>"
  BS/29 -> ToWs_Req_Bus_Sig29/1  "<testSig_CoETS_stCurrLimActive>"
  BS/30 -> ToWs_Req_Bus_Sig30/1  "<testSig_CoETS_trqInrCurrLim>"
  BS/31 -> ToWs_Req_Bus_Sig31/1  "<testSig_CoETS_trqInrVehLimMin_mp>"
  BS/32 -> ToWs_Req_Bus_Sig32/1  "<testSig_CoETS_rTrq>"
  BS/33 -> ToWs_Req_Bus_Sig33/1  "<testSig_CoETS_rTrqVMD>"
  BS/34 -> ToWs_Req_Bus_Sig34/1  "<testSig_CoETS_stLimInfo>"
  sig_Result_Bus/1 -> BS_Result/1, specifyOutputs/2(sig_Result_Bus)
  BS_Result/1 -> ToWs_Result_Bus_Sig1/1  "<CoETS_bLimInfo_DSM>"
  BS_Result/2 -> ToWs_Result_Bus_Sig2/1  "<CoETS_stCurrLim>"
  BS_Result/3 -> ToWs_Result_Bus_Sig3/1  "<CoETS_stCurrLimActive>"
  BS_Result/4 -> ToWs_Result_Bus_Sig4/1  "<CoETS_trqInrCurrLim>"
  BS_Result/5 -> ToWs_Result_Bus_Sig5/1  "<CoETS_trqInrVehLimMin_mp>"
  BS_Result/6 -> ToWs_Result_Bus_Sig6/1  "<CoETS_rTrq>"
  BS_Result/7 -> ToWs_Result_Bus_Sig7/1  "<CoETS_rTrqVMD>"
  BS_Result/8 -> ToWs_Result_Bus_Sig8/1  "<CoETS_stLimInfo>"
  specifyOutputs/1(result) -> result/1

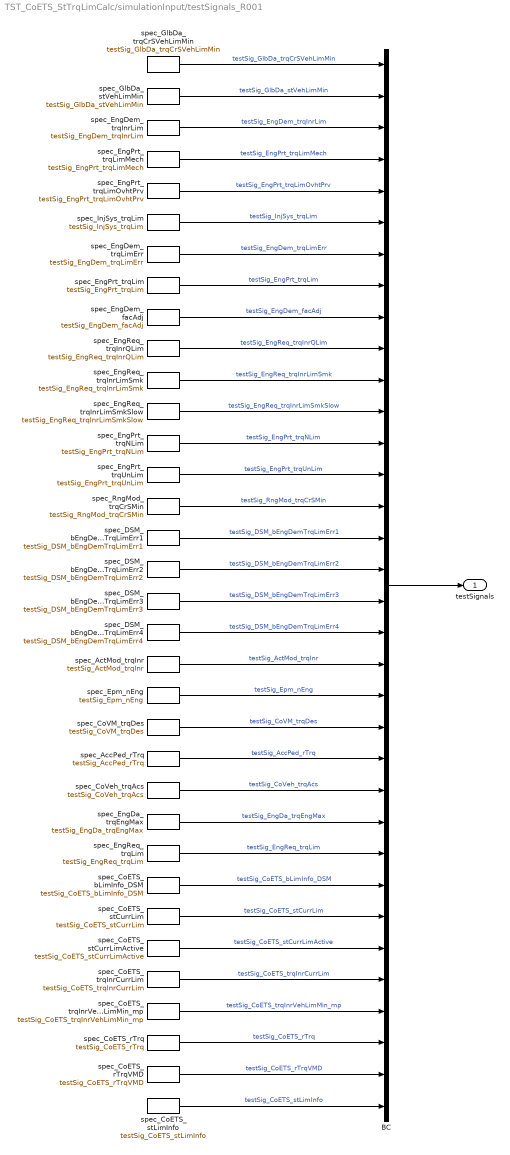
== system TST_CoETS_StTrqLimCalc/simulationInput/testSignals_R001 ==
  BC : BusCreator  Inputs=34
  spec_AccPed_rTrq : FromWorkspace  VariableName=testSig_AccPed_rTrq  Interpolate=off  OutputAfterFinalValue=Holding final value
  spec_ActMod_trqInr : FromWorkspace  VariableName=testSig_ActMod_trqInr  Interpolate=off  OutputAfterFinalValue=Holding final value
  spec_CoETS_bLimInfo_DSM : FromWorkspace  VariableName=testSig_CoETS_bLimInfo_DSM  Interpolate=off  OutputAfterFinalValue=Holding final value
  spec_CoETS_rTrq : FromWorkspace  VariableName=testSig_CoETS_rTrq  Interpolate=off  OutputAfterFinalValue=Holding final value
  spec_CoETS_rTrqVMD : FromWorkspace  VariableName=testSig_CoETS_rTrqVMD  Interpolate=off  OutputAfterFinalValue=Holding final value
  spec_CoETS_stCurrLim : FromWorkspace  VariableName=testSig_CoETS_stCurrLim  Interpolate=off  OutputAfterFinalValue=Holding final value
  spec_CoETS_stCurrLimActive : FromWorkspace  VariableName=testSig_CoETS_stCurrLimActive  Interpolate=off  OutputAfterFinalValue=Holding final value
  spec_CoETS_stLimInfo : FromWorkspace  VariableName=testSig_CoETS_stLimInfo  Interpolate=off  OutputAfterFinalValue=Holding final value
  spec_CoETS_trqInrCurrLim : FromWorkspace  VariableName=testSig_CoETS_trqInrCurrLim  Interpolate=off  OutputAfterFinalValue=Holding final value
  spec_CoETS_trqInrVehLimMin_mp : FromWorkspace  VariableName=testSig_CoETS_trqInrVehLimMin_mp  Interpolate=off  OutputAfterFinalValue=Holding final value
  spec_CoVM_trqDes : FromWorkspace  VariableName=testSig_CoVM_trqDes  Interpolate=off  OutputAfterFinalValue=Holding final value
  spec_CoVeh_trqAcs : FromWorkspace  VariableName=testSig_CoVeh_trqAcs  Interpolate=off  OutputAfterFinalValue=Holding final value
  spec_DSM_bEngDemTrqLimErr1 : FromWorkspace  VariableName=testSig_DSM_bEngDemTrqLimErr1  Interpolate=off  OutputAfterFinalValue=Holding final value
  spec_DSM_bEngDemTrqLimErr2 : FromWorkspace  VariableName=testSig_DSM_bEngDemTrqLimErr2  Interpolate=off  OutputAfterFinalValue=Holding final value
  spec_DSM_bEngDemTrqLimErr3 : FromWorkspace  VariableName=testSig_DSM_bEngDemTrqLimErr3  Interpolate=off  OutputAfterFinalValue=Holding final value
  spec_DSM_bEngDemTrqLimErr4 : FromWorkspace  VariableName=testSig_DSM_bEngDemTrqLimErr4  Interpolate=off  OutputAfterFinalValue=Holding final value
  spec_EngDa_trqEngMax : FromWorkspace  VariableName=testSig_EngDa_trqEngMax  Interpolate=off  OutputAfterFinalValue=Holding final value
  spec_EngDem_facAdj : FromWorkspace  VariableName=testSig_EngDem_facAdj  Interpolate=off  OutputAfterFinalValue=Holding final value
  spec_EngDem_trqInrLim : FromWorkspace  VariableName=testSig_EngDem_trqInrLim  Interpolate=off  OutputAfterFinalValue=Holding final value
  spec_EngDem_trqLimErr : FromWorkspace  VariableName=testSig_EngDem_trqLimErr  Interpolate=off  OutputAfterFinalValue=Holding final value
  spec_EngPrt_trqLim : FromWorkspace  VariableName=testSig_EngPrt_trqLim  Interpolate=off  OutputAfterFinalValue=Holding final value
  spec_EngPrt_trqLimMech : FromWorkspace  VariableName=testSig_EngPrt_trqLimMech  Interpolate=off  OutputAfterFinalValue=Holding final value
  spec_EngPrt_trqLimOvhtPrv : FromWorkspace  VariableName=testSig_EngPrt_trqLimOvhtPrv  Interpolate=off  OutputAfterFinalValue=Holding final value
  spec_EngPrt_trqNLim : FromWorkspace  VariableName=testSig_EngPrt_trqNLim  Interpolate=off  OutputAfterFinalValue=Holding final value
  spec_EngPrt_trqUnLim : FromWorkspace  VariableName=testSig_EngPrt_trqUnLim  Interpolate=off  OutputAfterFinalValue=Holding final value
  spec_EngReq_trqInrLimSmk : FromWorkspace  VariableName=testSig_EngReq_trqInrLimSmk  Interpolate=off  OutputAfterFinalValue=Holding final value
  spec_EngReq_trqInrLimSmkSlow : FromWorkspace  VariableName=testSig_EngReq_trqInrLimSmkSlow  Interpolate=off  OutputAfterFinalValue=Holding final value
  spec_EngReq_trqInrQLim : FromWorkspace  VariableName=testSig_EngReq_trqInrQLim  Interpolate=off  OutputAfterFinalValue=Holding final value
  spec_EngReq_trqLim : FromWorkspace  VariableName=testSig_EngReq_trqLim  Interpolate=off  OutputAfterFinalValue=Holding final value
  spec_Epm_nEng : FromWorkspace  VariableName=testSig_Epm_nEng  Interpolate=off  OutputAfterFinalValue=Holding final value
  spec_GlbDa_stVehLimMin : FromWorkspace  VariableName=testSig_GlbDa_stVehLimMin  Interpolate=off  OutputAfterFinalValue=Holding final value
  spec_GlbDa_trqCrSVehLimMin : FromWorkspace  VariableName=testSig_GlbDa_trqCrSVehLimMin  Interpolate=off  OutputAfterFinalValue=Holding final value
  spec_InjSys_trqLim : FromWorkspace  VariableName=testSig_InjSys_trqLim  Interpolate=off  OutputAfterFinalValue=Holding final value
  spec_RngMod_trqCrSMin : FromWorkspace  VariableName=testSig_RngMod_trqCrSMin  Interpolate=off  OutputAfterFinalValue=Holding final value
  testSignals : Outport
  wires:
  BC/1 -> testSignals/1
  spec_GlbDa_trqCrSVehLimMin/1 -> BC/1  "testSig_GlbDa_trqCrSVehLimMin"
  spec_GlbDa_stVehLimMin/1 -> BC/2  "testSig_GlbDa_stVehLimMin"
  spec_EngDem_trqInrLim/1 -> BC/3  "testSig_EngDem_trqInrLim"
  spec_EngPrt_trqLimMech/1 -> BC/4  "testSig_EngPrt_trqLimMech"
  spec_EngPrt_trqLimOvhtPrv/1 -> BC/5  "testSig_EngPrt_trqLimOvhtPrv"
  spec_InjSys_trqLim/1 -> BC/6  "testSig_InjSys_trqLim"
  spec_EngDem_trqLimErr/1 -> BC/7  "testSig_EngDem_trqLimErr"
  spec_EngPrt_trqLim/1 -> BC/8  "testSig_EngPrt_trqLim"
  spec_EngDem_facAdj/1 -> BC/9  "testSig_EngDem_facAdj"
  spec_EngReq_trqInrQLim/1 -> BC/10  "testSig_EngReq_trqInrQLim"
  spec_EngReq_trqInrLimSmk/1 -> BC/11  "testSig_EngReq_trqInrLimSmk"
  spec_EngReq_trqInrLimSmkSlow/1 -> BC/12  "testSig_EngReq_trqInrLimSmkSlow"
  spec_EngPrt_trqNLim/1 -> BC/13  "testSig_EngPrt_trqNLim"
  spec_EngPrt_trqUnLim/1 -> BC/14  "testSig_EngPrt_trqUnLim"
  spec_RngMod_trqCrSMin/1 -> BC/15  "testSig_RngMod_trqCrSMin"
  spec_DSM_bEngDemTrqLimErr1/1 -> BC/16  "testSig_DSM_bEngDemTrqLimErr1"
  spec_DSM_bEngDemTrqLimErr2/1 -> BC/17  "testSig_DSM_bEngDemTrqLimErr2"
  spec_DSM_bEngDemTrqLimErr3/1 -> BC/18  "testSig_DSM_bEngDemTrqLimErr3"
  spec_DSM_bEngDemTrqLimErr4/1 -> BC/19  "testSig_DSM_bEngDemTrqLimErr4"
  spec_ActMod_trqInr/1 -> BC/20  "testSig_ActMod_trqInr"
  spec_Epm_nEng/1 -> BC/21  "testSig_Epm_nEng"
  spec_CoVM_trqDes/1 -> BC/22  "testSig_CoVM_trqDes"
  spec_AccPed_rTrq/1 -> BC/23  "testSig_AccPed_rTrq"
  spec_CoVeh_trqAcs/1 -> BC/24  "testSig_CoVeh_trqAcs"
  spec_EngDa_trqEngMax/1 -> BC/25  "testSig_EngDa_trqEngMax"
  spec_EngReq_trqLim/1 -> BC/26  "testSig_EngReq_trqLim"
  spec_CoETS_bLimInfo_DSM/1 -> BC/27  "testSig_CoETS_bLimInfo_DSM"
  spec_CoETS_stCurrLim/1 -> BC/28  "testSig_CoETS_stCurrLim"
  spec_CoETS_stCurrLimActive/1 -> BC/29  "testSig_CoETS_stCurrLimActive"
  spec_CoETS_trqInrCurrLim/1 -> BC/30  "testSig_CoETS_trqInrCurrLim"
  spec_CoETS_trqInrVehLimMin_mp/1 -> BC/31  "testSig_CoETS_trqInrVehLimMin_mp"
  spec_CoETS_rTrq/1 -> BC/32  "testSig_CoETS_rTrq"
  spec_CoETS_rTrqVMD/1 -> BC/33  "testSig_CoETS_rTrqVMD"
  spec_CoETS_stLimInfo/1 -> BC/34  "testSig_CoETS_stLimInfo"

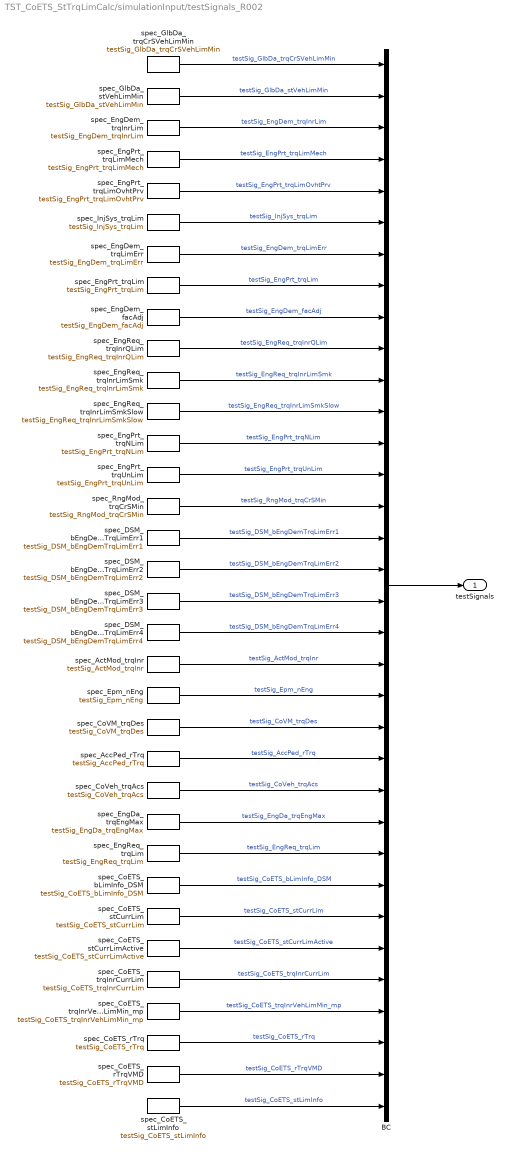
== system TST_CoETS_StTrqLimCalc/simulationInput/testSignals_R002 ==
  BC : BusCreator  Inputs=34
  spec_AccPed_rTrq : FromWorkspace  VariableName=testSig_AccPed_rTrq  Interpolate=off  OutputAfterFinalValue=Holding final value
  spec_ActMod_trqInr : FromWorkspace  VariableName=testSig_ActMod_trqInr  Interpolate=off  OutputAfterFinalValue=Holding final value
  spec_CoETS_bLimInfo_DSM : FromWorkspace  VariableName=testSig_CoETS_bLimInfo_DSM  Interpolate=off  OutputAfterFinalValue=Holding final value
  spec_CoETS_rTrq : FromWorkspace  VariableName=testSig_CoETS_rTrq  Interpolate=off  OutputAfterFinalValue=Holding final value
  spec_CoETS_rTrqVMD : FromWorkspace  VariableName=testSig_CoETS_rTrqVMD  Interpolate=off  OutputAfterFinalValue=Holding final value
  spec_CoETS_stCurrLim : FromWorkspace  VariableName=testSig_CoETS_stCurrLim  Interpolate=off  OutputAfterFinalValue=Holding final value
  spec_CoETS_stCurrLimActive : FromWorkspace  VariableName=testSig_CoETS_stCurrLimActive  Interpolate=off  OutputAfterFinalValue=Holding final value
  spec_CoETS_stLimInfo : FromWorkspace  VariableName=testSig_CoETS_stLimInfo  Interpolate=off  OutputAfterFinalValue=Holding final value
  spec_CoETS_trqInrCurrLim : FromWorkspace  VariableName=testSig_CoETS_trqInrCurrLim  Interpolate=off  OutputAfterFinalValue=Holding final value
  spec_CoETS_trqInrVehLimMin_mp : FromWorkspace  VariableName=testSig_CoETS_trqInrVehLimMin_mp  Interpolate=off  OutputAfterFinalValue=Holding final value
  spec_CoVM_trqDes : FromWorkspace  VariableName=testSig_CoVM_trqDes  Interpolate=off  OutputAfterFinalValue=Holding final value
  spec_CoVeh_trqAcs : FromWorkspace  VariableName=testSig_CoVeh_trqAcs  Interpolate=off  OutputAfterFinalValue=Holding final value
  spec_DSM_bEngDemTrqLimErr1 : FromWorkspace  VariableName=testSig_DSM_bEngDemTrqLimErr1  Interpolate=off  OutputAfterFinalValue=Holding final value
  spec_DSM_bEngDemTrqLimErr2 : FromWorkspace  VariableName=testSig_DSM_bEngDemTrqLimErr2  Interpolate=off  OutputAfterFinalValue=Holding final value
  spec_DSM_bEngDemTrqLimErr3 : FromWorkspace  VariableName=testSig_DSM_bEngDemTrqLimErr3  Interpolate=off  OutputAfterFinalValue=Holding final value
  spec_DSM_bEngDemTrqLimErr4 : FromWorkspace  VariableName=testSig_DSM_bEngDemTrqLimErr4  Interpolate=off  OutputAfterFinalValue=Holding final value
  spec_EngDa_trqEngMax : FromWorkspace  VariableName=testSig_EngDa_trqEngMax  Interpolate=off  OutputAfterFinalValue=Holding final value
  spec_EngDem_facAdj : FromWorkspace  VariableName=testSig_EngDem_facAdj  Interpolate=off  OutputAfterFinalValue=Holding final value
  spec_EngDem_trqInrLim : FromWorkspace  VariableName=testSig_EngDem_trqInrLim  Interpolate=off  OutputAfterFinalValue=Holding final value
  spec_EngDem_trqLimErr : FromWorkspace  VariableName=testSig_EngDem_trqLimErr  Interpolate=off  OutputAfterFinalValue=Holding final value
  spec_EngPrt_trqLim : FromWorkspace  VariableName=testSig_EngPrt_trqLim  Interpolate=off  OutputAfterFinalValue=Holding final value
  spec_EngPrt_trqLimMech : FromWorkspace  VariableName=testSig_EngPrt_trqLimMech  Interpolate=off  OutputAfterFinalValue=Holding final value
  spec_EngPrt_trqLimOvhtPrv : FromWorkspace  VariableName=testSig_EngPrt_trqLimOvhtPrv  Interpolate=off  OutputAfterFinalValue=Holding final value
  spec_EngPrt_trqNLim : FromWorkspace  VariableName=testSig_EngPrt_trqNLim  Interpolate=off  OutputAfterFinalValue=Holding final value
  spec_EngPrt_trqUnLim : FromWorkspace  VariableName=testSig_EngPrt_trqUnLim  Interpolate=off  OutputAfterFinalValue=Holding final value
  spec_EngReq_trqInrLimSmk : FromWorkspace  VariableName=testSig_EngReq_trqInrLimSmk  Interpolate=off  OutputAfterFinalValue=Holding final value
  spec_EngReq_trqInrLimSmkSlow : FromWorkspace  VariableName=testSig_EngReq_trqInrLimSmkSlow  Interpolate=off  OutputAfterFinalValue=Holding final value
  spec_EngReq_trqInrQLim : FromWorkspace  VariableName=testSig_EngReq_trqInrQLim  Interpolate=off  OutputAfterFinalValue=Holding final value
  spec_EngReq_trqLim : FromWorkspace  VariableName=testSig_EngReq_trqLim  Interpolate=off  OutputAfterFinalValue=Holding final value
  spec_Epm_nEng : FromWorkspace  VariableName=testSig_Epm_nEng  Interpolate=off  OutputAfterFinalValue=Holding final value
  spec_GlbDa_stVehLimMin : FromWorkspace  VariableName=testSig_GlbDa_stVehLimMin  Interpolate=off  OutputAfterFinalValue=Holding final value
  spec_GlbDa_trqCrSVehLimMin : FromWorkspace  VariableName=testSig_GlbDa_trqCrSVehLimMin  Interpolate=off  OutputAfterFinalValue=Holding final value
  spec_InjSys_trqLim : FromWorkspace  VariableName=testSig_InjSys_trqLim  Interpolate=off  OutputAfterFinalValue=Holding final value
  spec_RngMod_trqCrSMin : FromWorkspace  VariableName=testSig_RngMod_trqCrSMin  Interpolate=off  OutputAfterFinalValue=Holding final value
  testSignals : Outport
  wires:
  BC/1 -> testSignals/1
  spec_GlbDa_trqCrSVehLimMin/1 -> BC/1  "testSig_GlbDa_trqCrSVehLimMin"
  spec_GlbDa_stVehLimMin/1 -> BC/2  "testSig_GlbDa_stVehLimMin"
  spec_EngDem_trqInrLim/1 -> BC/3  "testSig_EngDem_trqInrLim"
  spec_EngPrt_trqLimMech/1 -> BC/4  "testSig_EngPrt_trqLimMech"
  spec_EngPrt_trqLimOvhtPrv/1 -> BC/5  "testSig_EngPrt_trqLimOvhtPrv"
  spec_InjSys_trqLim/1 -> BC/6  "testSig_InjSys_trqLim"
  spec_EngDem_trqLimErr/1 -> BC/7  "testSig_EngDem_trqLimErr"
  spec_EngPrt_trqLim/1 -> BC/8  "testSig_EngPrt_trqLim"
  spec_EngDem_facAdj/1 -> BC/9  "testSig_EngDem_facAdj"
  spec_EngReq_trqInrQLim/1 -> BC/10  "testSig_EngReq_trqInrQLim"
  spec_EngReq_trqInrLimSmk/1 -> BC/11  "testSig_EngReq_trqInrLimSmk"
  spec_EngReq_trqInrLimSmkSlow/1 -> BC/12  "testSig_EngReq_trqInrLimSmkSlow"
  spec_EngPrt_trqNLim/1 -> BC/13  "testSig_EngPrt_trqNLim"
  spec_EngPrt_trqUnLim/1 -> BC/14  "testSig_EngPrt_trqUnLim"
  spec_RngMod_trqCrSMin/1 -> BC/15  "testSig_RngMod_trqCrSMin"
  spec_DSM_bEngDemTrqLimErr1/1 -> BC/16  "testSig_DSM_bEngDemTrqLimErr1"
  spec_DSM_bEngDemTrqLimErr2/1 -> BC/17  "testSig_DSM_bEngDemTrqLimErr2"
  spec_DSM_bEngDemTrqLimErr3/1 -> BC/18  "testSig_DSM_bEngDemTrqLimErr3"
  spec_DSM_bEngDemTrqLimErr4/1 -> BC/19  "testSig_DSM_bEngDemTrqLimErr4"
  spec_ActMod_trqInr/1 -> BC/20  "testSig_ActMod_trqInr"
  spec_Epm_nEng/1 -> BC/21  "testSig_Epm_nEng"
  spec_CoVM_trqDes/1 -> BC/22  "testSig_CoVM_trqDes"
  spec_AccPed_rTrq/1 -> BC/23  "testSig_AccPed_rTrq"
  spec_CoVeh_trqAcs/1 -> BC/24  "testSig_CoVeh_trqAcs"
  spec_EngDa_trqEngMax/1 -> BC/25  "testSig_EngDa_trqEngMax"
  spec_EngReq_trqLim/1 -> BC/26  "testSig_EngReq_trqLim"
  spec_CoETS_bLimInfo_DSM/1 -> BC/27  "testSig_CoETS_bLimInfo_DSM"
  spec_CoETS_stCurrLim/1 -> BC/28  "testSig_CoETS_stCurrLim"
  spec_CoETS_stCurrLimActive/1 -> BC/29  "testSig_CoETS_stCurrLimActive"
  spec_CoETS_trqInrCurrLim/1 -> BC/30  "testSig_CoETS_trqInrCurrLim"
  spec_CoETS_trqInrVehLimMin_mp/1 -> BC/31  "testSig_CoETS_trqInrVehLimMin_mp"
  spec_CoETS_rTrq/1 -> BC/32  "testSig_CoETS_rTrq"
  spec_CoETS_rTrqVMD/1 -> BC/33  "testSig_CoETS_rTrqVMD"
  spec_CoETS_stLimInfo/1 -> BC/34  "testSig_CoETS_stLimInfo"

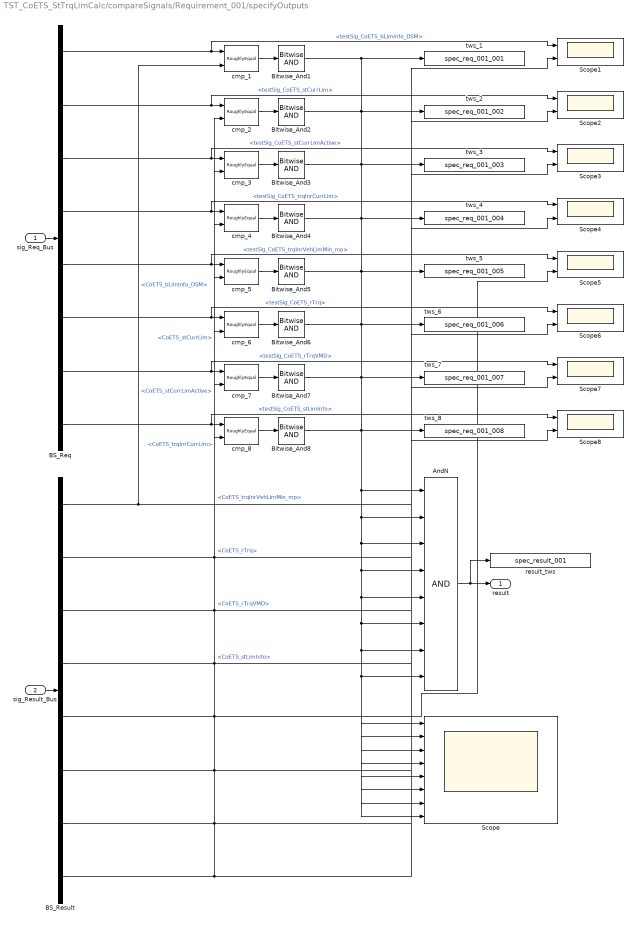
== system TST_CoETS_StTrqLimCalc/compareSignals/Requirement_001/specifyOutputs ==
  sig_Req_Bus : Inport
  sig_Result_Bus : Inport  Port=2
  AndN : Logic  Inputs=8
  BS_Req : BusSelector  OutputSignals=testSig_CoETS_bLimInfo_DSM,testSig_CoETS_stCurrLim,testSig_CoETS_stCurrLimActive,testSig_CoETS_trqInrCurrLim,testSig_CoETS_trqInrVehLimMin_mp,testSig_CoETS_rTrq,testSig_CoETS_rTrqVMD,testSig_CoETS_stLimInfo
  BS_Result : BusSelector  OutputSignals=CoETS_bLimInfo_DSM,CoETS_stCurrLim,CoETS_stCurrLimActive,CoETS_trqInrCurrLim,CoETS_trqInrVehLimMin_mp,CoETS_rTrq,CoETS_rTrqVMD,CoETS_stLimInfo
  Bitwise_And{1..8} (8 alike) : simulink/Logic and Bit Operations/Bitwise Operator  logicop=AND  UseBitMask=off  BitMask=bin2dec('11011001')  BitMaskRealWorld=Stored Integer
  Scope : Scope  NumInputPorts=8
  Scope{1..8} (8 alike) : Scope  NumInputPorts=2
  cmp_{1..5,8} (6 alike) : UnitTest_Lib/RoughlyEqual  slope=0.1
  cmp_6 : UnitTest_Lib/RoughlyEqual  slope=5
  cmp_7 : UnitTest_Lib/RoughlyEqual  slope=20
  result_tws : ToWorkspace  VariableName=spec_result_001
  tws_1 : ToWorkspace  VariableName=spec_req_001_001
  tws_2 : ToWorkspace  VariableName=spec_req_001_002
  tws_3 : ToWorkspace  VariableName=spec_req_001_003
  tws_4 : ToWorkspace  VariableName=spec_req_001_004
  tws_5 : ToWorkspace  VariableName=spec_req_001_005
  tws_6 : ToWorkspace  VariableName=spec_req_001_006
  tws_7 : ToWorkspace  VariableName=spec_req_001_007
  tws_8 : ToWorkspace  VariableName=spec_req_001_008
  result : Outport
  wires:
  sig_Req_Bus/1 -> BS_Req/1
  sig_Result_Bus/1 -> BS_Result/1
  AndN/1 -> result/1, result_tws/1
  BS_Req/1 -> cmp_1/1, Scope1/1  "<testSig_CoETS_bLimInfo_DSM>"
  BS_Result/1 -> cmp_1/2, Scope1/2  "<CoETS_bLimInfo_DSM>"
  cmp_1/1 -> Bitwise_And1/1
  Bitwise_And1/1 -> AndN/1, Scope/1, tws_1/1
  BS_Req/2 -> cmp_2/1, Scope2/1  "<testSig_CoETS_stCurrLim>"
  BS_Result/2 -> cmp_2/2, Scope2/2  "<CoETS_stCurrLim>"
  cmp_2/1 -> Bitwise_And2/1
  Bitwise_And2/1 -> AndN/2, Scope/2, tws_2/1
  BS_Req/3 -> cmp_3/1, Scope3/1  "<testSig_CoETS_stCurrLimActive>"
  BS_Result/3 -> cmp_3/2, Scope3/2  "<CoETS_stCurrLimActive>"
  cmp_3/1 -> Bitwise_And3/1
  Bitwise_And3/1 -> AndN/3, Scope/3, tws_3/1
  BS_Req/4 -> cmp_4/1, Scope4/1  "<testSig_CoETS_trqInrCurrLim>"
  BS_Result/4 -> cmp_4/2, Scope4/2  "<CoETS_trqInrCurrLim>"
  cmp_4/1 -> Bitwise_And4/1
  Bitwise_And4/1 -> AndN/4, Scope/4, tws_4/1
  BS_Req/5 -> cmp_5/1, Scope5/1  "<testSig_CoETS_trqInrVehLimMin_mp>"
  BS_Result/5 -> cmp_5/2, Scope5/2  "<CoETS_trqInrVehLimMin_mp>"
  cmp_5/1 -> Bitwise_And5/1
  Bitwise_And5/1 -> AndN/5, Scope/5, tws_5/1
  BS_Req/6 -> cmp_6/1, Scope6/1  "<testSig_CoETS_rTrq>"
  BS_Result/6 -> cmp_6/2, Scope6/2  "<CoETS_rTrq>"
  cmp_6/1 -> Bitwise_And6/1
  Bitwise_And6/1 -> AndN/6, Scope/6, tws_6/1
  BS_Req/7 -> cmp_7/1, Scope7/1  "<testSig_CoETS_rTrqVMD>"
  BS_Result/7 -> cmp_7/2, Scope7/2  "<CoETS_rTrqVMD>"
  cmp_7/1 -> Bitwise_And7/1
  Bitwise_And7/1 -> AndN/7, Scope/7, tws_7/1
  BS_Req/8 -> cmp_8/1, Scope8/1  "<testSig_CoETS_stLimInfo>"
  BS_Result/8 -> cmp_8/2, Scope8/2  "<CoETS_stLimInfo>"
  cmp_8/1 -> Bitwise_And8/1
  Bitwise_And8/1 -> AndN/8, Scope/8, tws_8/1

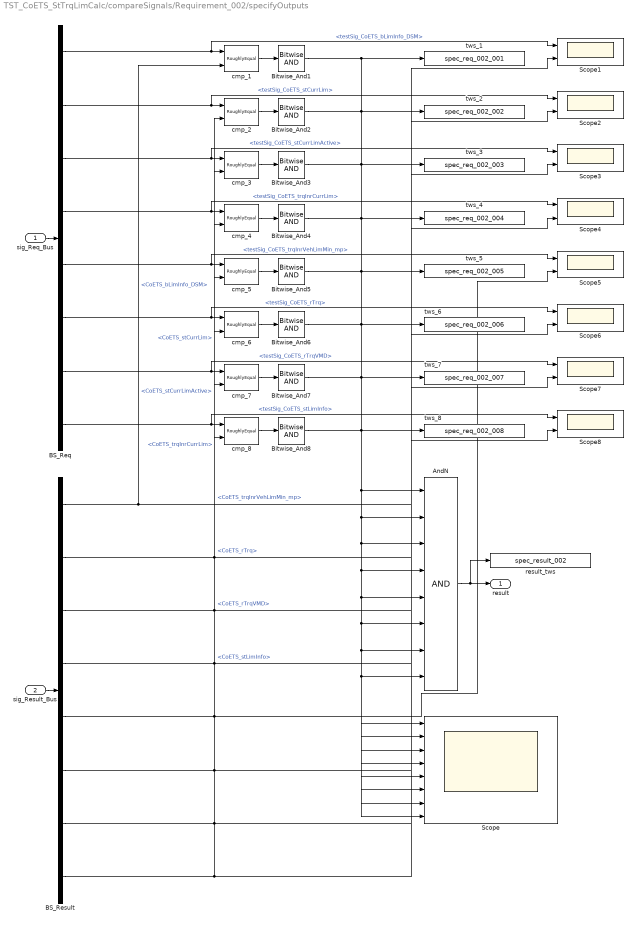
== system TST_CoETS_StTrqLimCalc/compareSignals/Requirement_002/specifyOutputs ==
  sig_Req_Bus : Inport
  sig_Result_Bus : Inport  Port=2
  AndN : Logic  Inputs=8
  BS_Req : BusSelector  OutputSignals=testSig_CoETS_bLimInfo_DSM,testSig_CoETS_stCurrLim,testSig_CoETS_stCurrLimActive,testSig_CoETS_trqInrCurrLim,testSig_CoETS_trqInrVehLimMin_mp,testSig_CoETS_rTrq,testSig_CoETS_rTrqVMD,testSig_CoETS_stLimInfo
  BS_Result : BusSelector  OutputSignals=CoETS_bLimInfo_DSM,CoETS_stCurrLim,CoETS_stCurrLimActive,CoETS_trqInrCurrLim,CoETS_trqInrVehLimMin_mp,CoETS_rTrq,CoETS_rTrqVMD,CoETS_stLimInfo
  Bitwise_And{1..8} (8 alike) : simulink/Logic and Bit Operations/Bitwise Operator  logicop=AND  UseBitMask=off  BitMask=bin2dec('11011001')  BitMaskRealWorld=Stored Integer
  Scope : Scope  NumInputPorts=8
  Scope{1..8} (8 alike) : Scope  NumInputPorts=2
  cmp_{1..6,8} (7 alike) : UnitTest_Lib/RoughlyEqual  slope=0.1
  cmp_7 : UnitTest_Lib/RoughlyEqual  slope=20
  result_tws : ToWorkspace  VariableName=spec_result_002
  tws_1 : ToWorkspace  VariableName=spec_req_002_001
  tws_2 : ToWorkspace  VariableName=spec_req_002_002
  tws_3 : ToWorkspace  VariableName=spec_req_002_003
  tws_4 : ToWorkspace  VariableName=spec_req_002_004
  tws_5 : ToWorkspace  VariableName=spec_req_002_005
  tws_6 : ToWorkspace  VariableName=spec_req_002_006
  tws_7 : ToWorkspace  VariableName=spec_req_002_007
  tws_8 : ToWorkspace  VariableName=spec_req_002_008
  result : Outport
  wires:
  sig_Req_Bus/1 -> BS_Req/1
  sig_Result_Bus/1 -> BS_Result/1
  AndN/1 -> result/1, result_tws/1
  BS_Req/1 -> cmp_1/1, Scope1/1  "<testSig_CoETS_bLimInfo_DSM>"
  BS_Result/1 -> cmp_1/2, Scope1/2  "<CoETS_bLimInfo_DSM>"
  cmp_1/1 -> Bitwise_And1/1
  Bitwise_And1/1 -> AndN/1, Scope/1, tws_1/1
  BS_Req/2 -> cmp_2/1, Scope2/1  "<testSig_CoETS_stCurrLim>"
  BS_Result/2 -> cmp_2/2, Scope2/2  "<CoETS_stCurrLim>"
  cmp_2/1 -> Bitwise_And2/1
  Bitwise_And2/1 -> AndN/2, Scope/2, tws_2/1
  BS_Req/3 -> cmp_3/1, Scope3/1  "<testSig_CoETS_stCurrLimActive>"
  BS_Result/3 -> cmp_3/2, Scope3/2  "<CoETS_stCurrLimActive>"
  cmp_3/1 -> Bitwise_And3/1
  Bitwise_And3/1 -> AndN/3, Scope/3, tws_3/1
  BS_Req/4 -> cmp_4/1, Scope4/1  "<testSig_CoETS_trqInrCurrLim>"
  BS_Result/4 -> cmp_4/2, Scope4/2  "<CoETS_trqInrCurrLim>"
  cmp_4/1 -> Bitwise_And4/1
  Bitwise_And4/1 -> AndN/4, Scope/4, tws_4/1
  BS_Req/5 -> cmp_5/1, Scope5/1  "<testSig_CoETS_trqInrVehLimMin_mp>"
  BS_Result/5 -> cmp_5/2, Scope5/2  "<CoETS_trqInrVehLimMin_mp>"
  cmp_5/1 -> Bitwise_And5/1
  Bitwise_And5/1 -> AndN/5, Scope/5, tws_5/1
  BS_Req/6 -> cmp_6/1, Scope6/1  "<testSig_CoETS_rTrq>"
  BS_Result/6 -> cmp_6/2, Scope6/2  "<CoETS_rTrq>"
  cmp_6/1 -> Bitwise_And6/1
  Bitwise_And6/1 -> AndN/6, Scope/6, tws_6/1
  BS_Req/7 -> cmp_7/1, Scope7/1  "<testSig_CoETS_rTrqVMD>"
  BS_Result/7 -> cmp_7/2, Scope7/2  "<CoETS_rTrqVMD>"
  cmp_7/1 -> Bitwise_And7/1
  Bitwise_And7/1 -> AndN/7, Scope/7, tws_7/1
  BS_Req/8 -> cmp_8/1, Scope8/1  "<testSig_CoETS_stLimInfo>"
  BS_Result/8 -> cmp_8/2, Scope8/2  "<CoETS_stLimInfo>"
  cmp_8/1 -> Bitwise_And8/1
  Bitwise_And8/1 -> AndN/8, Scope/8, tws_8/1
